simulink model "prob1"  (R2020b)
settings: Solver=VariableStepAuto  StartTime=0.0  StopTime=10.0  RelTol=1e-3
settings Model: Creator=nadee  LastModifiedBy=nadee

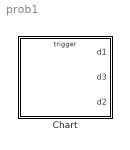
== system prob1 ==
  Chart : Stateflow chart  TreatAsAtomicUnit=on

== stateflow chart prob1/Chart ==
  state D1 [parallel]
    settings: executionOrder=1
    state Zero
      entry:d1=0;
    state One
      entry:d1=1;
    state Two
      entry:d1=2;
    state Four
      entry:d1=4;
    state Three
      entry:d1=3;
    (default) -> D1.Zero
    D1.Zero -> D1.One : InpClick
    D1.One -> D1.Two : InpClick
    D1.Four -> D1.Zero : InpClick/{D2.InC2;}
    D1.Two -> D1.Three : InpClick
    D1.Three -> D1.Four : InpClick
  state D2 [parallel]
    settings: executionOrder=2
    state Zero
      entry:d2=0;
    state One
      entry:d2=1;
    state Two
      entry:d2=2;
    state Four
      entry:d2=4;
    state Three
      entry:d2=3;
    (default) -> D2.Zero
    D2.Zero -> D2.One : InC2
    D2.One -> D2.Two : InC2
    D2.Four -> D2.Zero : InC2/{D3.InC3;}
    D2.Two -> D2.Three : InC2
    D2.Three -> D2.Four : InC2
  state D3 [parallel]
    settings: executionOrder=3
    state Zero
      entry:d3=0;
    state One
      entry:d3=1;
    state Two
      entry:d3=2;
    state Four
      entry:d3=4;
    state Three
      entry:d3=3;
    (default) -> D3.Zero
    D3.Zero -> D3.One : InC3
    D3.One -> D3.Two : InC3
    D3.Four -> D3.Zero : InC3
    D3.Two -> D3.Three : InC3
    D3.Three -> D3.Four : InC3
  data: d1 output; d3 output; d2 output
  events: InC2 local FUNCTION_CALL_EVENT; InC3 local FUNCTION_CALL_EVENT; InpClick input EITHER_EDGE_EVENT
